simulink library "discrete_timer"  (R2020a)
settings: Solver=ode45  StartTime=0.0  StopTime=10.0  RelTol=1e-3  EnableMultiTasking=on
libraries: simulink x1
settings Model: Creator=Harjot  LastModifiedBy=Harjot
settings DataIOCC: LimitDataPoints=on
settings OptimizationCC: LifeSpan=inf
settings DebuggingCC: AllowSymbolicDim=off  SFUnexpectedBacktrackingDiag=warning  SFNoUnconditionalDefaultTransitionDiag=warning  SFExecutionAtInitializationDiag=none  ArithmeticOperatorsInVariantConditions=warning
settings SFSimCC: SimUseLocalCustomCode=off  CustomCodeUndefinedFunction=UseInterfaceOnly
settings RTWCC: RTWUseLocalCustomCode=off
settings CodeAppCC: StateflowObjectComments=on
settings GRTTargetCC: TargetLangStandard=C89/C90 (ANSI)
settings ConfigComp: CovMetricSettings=dw  CovHtmlReporting=on  CovSaveCumulativeToWorkspaceVar=on  CovSaveSingleToWorkspaceVar=on  CovExternalEMLEnable=off

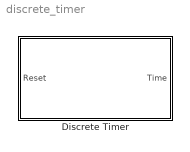
== system discrete_timer ==
  Discrete Timer : Subsystem
      mask DialogControl Container6 Prompt: Discrete Timer Block
      mask DialogControl Control3 Prompt: This block implements a timer with a reset

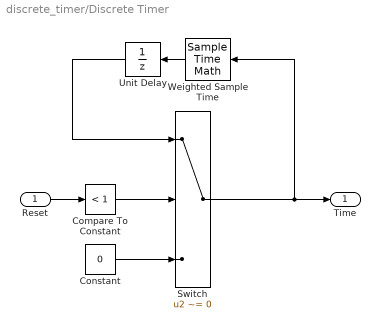
== system discrete_timer/Discrete Timer ==
  Reset : Inport
  Compare To Constant : simulink/Logic and Bit Operations/Compare To Constant  relop=<  const=1  OutDataTypeStr=boolean
  Constant : Constant  Value=0
  Switch : Switch  Criteria=u2 ~= 0
  Unit Delay : UnitDelay  SampleTime=-1  HasFrameUpgradeWarning=on
  Weighted Sample Time : SampleTimeMath
  Time : Outport  VectorParamsAs1DForOutWhenUnconnected=off
  wires:
  Weighted Sample Time/1 -> Unit Delay/1
  Constant/1 -> Switch/3
  Reset/1 -> Compare To Constant/1
  Compare To Constant/1 -> Switch/2
  Switch/1 -> Weighted Sample Time/1, Time/1
  Unit Delay/1 -> Switch/1
